simulink library "Mat2Quat"  (R2014b)
settings: Solver=ode45  StartTime=0.0  StopTime=10.0  RelTol=1e-3
settings Model: Creator=Hp  LastModifiedBy=Hp

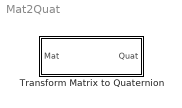
== system Mat2Quat ==
  Transform Matrix to Quaternion : Subsystem

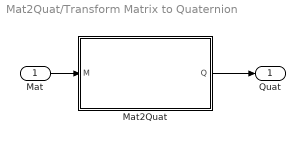
== system Mat2Quat/Transform Matrix to Quaternion ==
  Mat : Inport
  Mat2Quat : MATLAB Function  TreatAsAtomicUnit=on
  Quat : Outport
  wires:
  Mat2Quat/1(Q) -> Quat/1
  Mat/1 -> Mat2Quat/1(M)

== matlab function Mat2Quat/Transform Matrix to Quaternion/Mat2Quat ==
  data: M input; Q output
function Q=Mat2Quat(M)
% R1->R2 quaternion calculation corresponding to the TRANSFORM matrix M
% (transpose of change of basis matrix) from R1 to R2 (direct orthogonal)
% such that V[R2]=M*V[R1]
[~,I]=max(diag(M));  % Indice I du maximum de la diagonal de M
% I=I(1);
u=I; v=rem(I,3)+1; w=rem(I+1,3)+1; % Calcul des autres indices
r=sqrt(1+M(u,u)-M(v,v)-M(w,w));
Q=zeros(4,1);
if r==0
   Q=[1;0;0;0];
else
   Q(1)=M(v,w)-M(w,v); Q(u+1)=r^2; Q(v+1)=M(u,v)+M(v,u); Q(w+1)=M(w,u)+M(u,w);
end
Q=1/norm(Q)*Q;
end
